simulink model "px4_mc_sim_full_distrb_ekf"  (R2019b)
settings: Solver=FixedStepAuto  StartTime=0.0  StopTime=sim_time  FixedStep=1/sim_freq  RelTol=1e-3
values from neighbouring files (symbols this model uses):
  C_D = [0.064; 0.067; 0.089].*0    [full_distrb_model_parameters.m]    (also in model_parameters.m)
  d = 0.11    [full_distrb_model_parameters.m]    (also in model_parameters.m)
  hover_perc = m*g / max_total_T    [full_distrb_model_parameters.m]    (also in model_parameters.m)
  Ixx = 1.326e-3    (= 0.001326)    [full_distrb_model_parameters.m]    (also in model_parameters.m)
  Iyy = 9.3e-4    (= 0.00093)    [full_distrb_model_parameters.m]    (also in model_parameters.m)
  Izz = 1.95e-3    (= 0.00195)    [full_distrb_model_parameters.m]    (also in model_parameters.m)
  m = 0.66    [full_distrb_model_parameters.m]    (also in model_parameters.m)
  max_T = max_total_T / 4    [full_distrb_model_parameters.m]    (also in model_parameters.m)
  meas_noise = 0.000001    (= 1e-06)    [full_distrb_model_parameters.m]    (also in full_performance_analysis.m; model_parameters.m; noise_matrices.m = 0.0001; run_sim_full_dstrb.m)
  Pk_init = zeros(15)    [full_distrb_model_parameters.m]    (also in full_performance_analysis.m; model_parameters.m = zeros(12); noise_matrices.m = zeros(12,12); run_sim_full_dstrb.m)
  pos_e_step = [0,0,0]    [full_performance_analysis.m]    (also in performance_analysis.m; run_sim.m = [0,2,0]; run_sim_full_dstrb.m)
  pulse_amplitude = 0.1    [run_sim.m]    (also in run_sim_full_dstrb.m)
  pulse_period = 40    [run_sim.m]    (also in run_sim_full_dstrb.m)
  Qk = C22'*C12    [full_distrb_model_parameters.m]    (also in full_performance_analysis.m; model_parameters.m; noise_matrices.m; run_sim_full_dstrb.m)
  r_D = 7.997e-3    (= 0.007997)    [full_distrb_model_parameters.m]    (also in model_parameters.m)
  ramp_max = 0.15    [full_performance_analysis.m]    (also in performance_analysis.m; run_sim.m = 0.5; run_sim_full_dstrb.m = 0.1)
  ramp_slope = 0.05    [full_performance_analysis.m]    (also in performance_analysis.m; run_sim.m; run_sim_full_dstrb.m = 0.01)
  Rk = eye(9)*meas_noise    [full_distrb_model_parameters.m]    (also in full_performance_analysis.m; model_parameters.m; noise_matrices.m; run_sim_full_dstrb.m)
  sinus_amplitude = 0.2    [full_performance_analysis.m]    (also in performance_analysis.m; run_sim.m = 0.1; run_sim_full_dstrb.m = 0.1)
  sinus_bias = 0    [full_performance_analysis.m]    (also in performance_analysis.m; run_sim.m; run_sim_full_dstrb.m)
  sinus_freq = 3    [full_performance_analysis.m]    (also in performance_analysis.m = 5; run_sim.m = 1; run_sim_full_dstrb.m = 10)
  step_delay = 3    [full_performance_analysis.m]    (also in performance_analysis.m; run_sim.m = 1; run_sim_full_dstrb.m = 1)
  step_mag = 0.1    [full_performance_analysis.m]    (also in performance_analysis.m; run_sim.m = 0.5; run_sim_full_dstrb.m)
  tau_T = 0.002    [full_distrb_model_parameters.m]    (also in model_parameters.m)
  virtual_controls_mat = [1 1 1 1; -1/sqrt(2) 1/sqrt(2) 1/sqrt(2) -1/sqrt(2); 1/sqrt(2) -1/sqrt(2) 1/sqrt(2) -1/sqrt(2); 1 1 -1 -1]    [full_distrb_model_parameters.m]    (also in model_parameters.m)
  wind = [0; 0; 0]    [full_distrb_model_parameters.m]    (also in model_parameters.m)
  X_hat_init = zeros(15,1)    [full_distrb_model_parameters.m]    (also in full_performance_analysis.m; model_parameters.m = zeros(12,1); noise_matrices.m = zeros(12,1); run_sim_full_dstrb.m)
  yaw_step = 0    [full_performance_analysis.m]    (also in performance_analysis.m; run_sim.m; run_sim_full_dstrb.m)
undefined symbols (not defined in the file or in its folder): br_filt_denom, br_filt_num, DiscIntNeverNeededParam, eta_w, g, MC_PITCH_P, MC_PITCHRATE_D, MC_PITCHRATE_I, MC_PITCHRATE_MAX, MC_PITCHRATE_P, MC_PR_INT_LIM, MC_ROLL_P, MC_ROLLRATE_D, MC_ROLLRATE_I, MC_ROLLRATE_MAX, MC_ROLLRATE_P, MC_RR_INT_LIM, MC_YAW_P, MC_YAWRATE_D, MC_YAWRATE_I, MC_YAWRATE_MAX, MC_YAWRATE_P, MC_YR_INT_LIM, MPC_THR_MAX, MPC_THR_MIN, MPC_TILTMAX_AIR, MPC_XY_P, MPC_XY_VEL_D, MPC_XY_VEL_I, MPC_XY_VEL_MAX, MPC_XY_VEL_P, MPC_Z_P, MPC_Z_VEL_D, MPC_Z_VEL_I, MPC_Z_VEL_MAX_DN, MPC_Z_VEL_MAX_UP, MPC_Z_VEL_P, rho, sim_freq, vel_filt_denom, vel_filt_num
libraries: simulink x7, sharedtransform x3, shared6dof x1
(part 2 of 2)

== matlab function px4_mc_sim_full_distrb_ekf/Extended Kalman Filter/EKF ==
  data: yk input size=[1 9]; u input size=[4 1]; X_hat output size=[15 1]; x_hat_prev input size=[15, 1]; P_prev input size=[15 15]; Pk output size=[15 15]; Qk parameter size=[15 15]; Rk parameter size=[9 9]; m parameter; g parameter; Ixx parameter; Iyy parameter; Izz parameter; r_D parameter; d parameter
function [X_hat,Pk]= fcn(yk,u,x_hat_prev,P_prev,Qk, Rk,m, g, Ixx, Iyy, Izz, r_D, d)

U=x_hat_prev(1);
V=x_hat_prev(2);
W=x_hat_prev(3);
P=x_hat_prev(4);
Q=x_hat_prev(5);
R=x_hat_prev(6);
phi=x_hat_prev(7);
theta=x_hat_prev(8);
psi=x_hat_prev(9);
Fx=x_hat_prev(10);
Fy=x_hat_prev(11);
Fz=x_hat_prev(12);
Mx=x_hat_prev(13);
My=x_hat_prev(14);
Mz=x_hat_prev(15);
del_t=u(1);
del_a=u(2);
del_e=u(3);
del_r=u(4);

yk=yk';

F = @(U,V,W,P,Q,R,phi,theta,psi,del_t,del_a,del_e,del_r,Fx,Fy,Fz,Mx,My,Mz)[
[                            R*V - Q*W + (Fx - g*m*sin(theta))/m]
[                   P*W - R*U + (Fy + g*m*cos(theta)*sin(phi))/m]
[ Q*U - P*V + (Fz - del_t - d*del_a + g*m*cos(phi)*cos(theta))/m]
[                     (Mx + d*del_a)/Ixx + (Q*R*(Iyy - Izz))/Ixx]
[                     (My + d*del_e)/Iyy - (P*R*(Ixx - Izz))/Iyy]
[                   (Mz + del_r*r_D)/Izz + (P*Q*(Ixx - Izz))/Izz]
[              P + R*cos(phi)*tan(theta) + Q*sin(phi)*tan(theta)]
[                                        Q*cos(phi) - R*sin(phi)]
[              (R*cos(phi))/cos(theta) + (Q*sin(phi))/cos(theta)]
[                                                              0]
[                                                              0]
[                                                              0]
[                                                              0]
[                                                              0]
[                                                              0]
];
           
           
 %% Jacobian
 Fk = @(U,V,W,P,Q,R,phi,theta,psi,Fx,Fy,Fz) [
[      1,  R/250, -Q/250,                          0,                    -W/250,                      V/250,                                                             0,                                                                     -(g*cos(theta))/250, 0, 1/(250*m),         0,         0,           0,           0,           0]
[ -R/250,      1,  P/250,                      W/250,                         0,                     -U/250,                                   (g*cos(phi)*cos(theta))/250,                                                            -(g*sin(phi)*sin(theta))/250, 0,         0, 1/(250*m),         0,           0,           0,           0]
[  Q/250, -P/250,      1,                     -V/250,                     U/250,                          0,                                  -(g*cos(theta)*sin(phi))/250,                                                            -(g*cos(phi)*sin(theta))/250, 0,         0,         0, 1/(250*m),           0,           0,           0]
[      0,      0,      0,                          1, (R*(Iyy - Izz))/(250*Ixx),  (Q*(Iyy - Izz))/(250*Ixx),                                                             0,                                                                                       0, 0,         0,         0,         0, 1/(250*Ixx),           0,           0]
[      0,      0,      0, -(R*(Ixx - Izz))/(250*Iyy),                         1, -(P*(Ixx - Izz))/(250*Iyy),                                                             0,                                                                                       0, 0,         0,         0,         0,           0, 1/(250*Iyy),           0]
[      0,      0,      0,  (Q*(Ixx - Izz))/(250*Izz), (P*(Ixx - Izz))/(250*Izz),                          1,                                                             0,                                                                                       0, 0,         0,         0,         0,           0,           0, 1/(250*Izz)]
[      0,      0,      0,                      1/250, (sin(phi)*tan(theta))/250,  (cos(phi)*tan(theta))/250, (Q*cos(phi)*tan(theta))/250 - (R*sin(phi)*tan(theta))/250 + 1,               (R*cos(phi)*(tan(theta)^2 + 1))/250 + (Q*sin(phi)*(tan(theta)^2 + 1))/250, 0,         0,         0,         0,           0,           0,           0]
[      0,      0,      0,                          0,              cos(phi)/250,              -sin(phi)/250,                         - (R*cos(phi))/250 - (Q*sin(phi))/250,                                                                                       1, 0,         0,         0,         0,           0,           0,           0]
[      0,      0,      0,                          0, sin(phi)/(250*cos(theta)),  cos(phi)/(250*cos(theta)), (Q*cos(phi))/(250*cos(theta)) - (R*sin(phi))/(250*cos(theta)), (R*cos(phi)*sin(theta))/(250*cos(theta)^2) + (Q*sin(phi)*sin(theta))/(250*cos(theta)^2), 1,         0,         0,         0,           0,           0,           0]
[      0,      0,      0,                          0,                         0,                          0,                                                             0,                                                                                       0, 0,         1,         0,         0,           0,           0,           0]
[      0,      0,      0,                          0,                         0,                          0,                                                             0,                                                                                       0, 0,         0,         1,         0,           0,           0,           0]
[      0,      0,      0,                          0,                         0,                          0,                                                             0,                                                                                       0, 0,         0,         0,         1,           0,           0,           0]
[      0,      0,      0,                          0,                         0,                          0,                                                             0,                                                                                       0, 0,         0,         0,         0,           1,           0,           0]
[      0,      0,      0,                          0,                         0,                          0,                                                             0,                                                                                       0, 0,         0,         0,         0,           0,           1,           0]
[      0,      0,      0,                          0,                         0,                          0,                                                             0,                                                                                       0, 0,         0,         0,         0,           0,           0,           1]
];
%% Control Update
Pk_ =  Fk(U,V,W,P,Q,R,phi,theta,psi,Fx,Fy,Fz) * P_prev * transpose( Fk(U,V,W,P,Q,R,phi,theta,psi,Fx,Fy,Fz) ) + Qk;
Xk_ = x_hat_prev + F(U,V,W,P,Q,R,phi,theta,psi,del_t,del_a,del_e,del_r,Fx,Fy,Fz,Mx,My,Mz)*1/250; 
         
Hk = eye(9,15);
%% Measurement Update
Lk = Pk_*transpose(Hk)*inv(Hk*Pk_*transpose(Hk) + Rk);
Pk = (eye(15) - Lk*Hk)*Pk_;
X_hat = Xk_ + Lk*(yk - Hk*Xk_);
